simulink model "Project2_2"  (R2025b)
settings: Solver=VariableStepAuto  StartTime=0.0  StopTime=10.0  RelTol=1e-3
undefined symbols (not defined in the file or in its folder): A, F, Ti
settings Model: Creator=night  LastModifiedBy=night

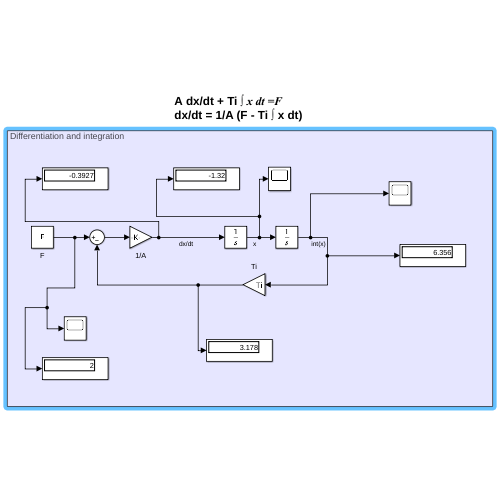
[thumbnail: Simulink's stored preview of the top-level diagram]
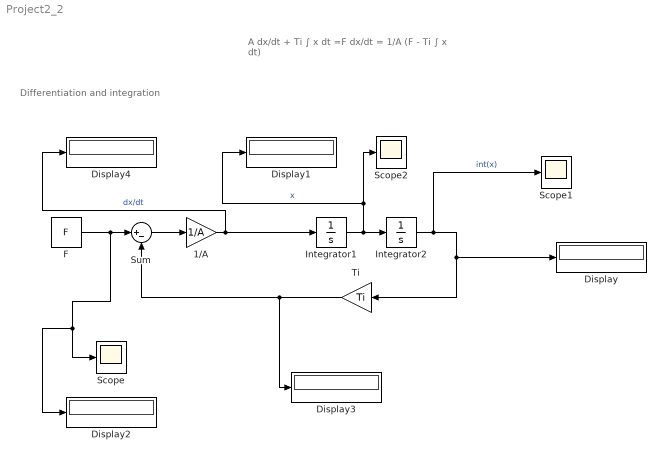
== system Project2_2 ==
  note: A dx/dt + Ti ∫ x dt =F
      | dx/dt = 1/A (F - Ti ∫ x dt)
  note: Differentiation and integration
  1/A : Gain  Gain=1/A
  Display{,1..4} (5 alike) : Display
  F : Constant  Value=F
  Integrator1 : Integrator
  Integrator2 : Integrator
  Scope : Scope
      settings: ActiveDisplayYMinimum=1  ActiveDisplayYMaximum=3
  Scope1 : Scope
      settings: ActiveDisplayYMinimum=-1  ActiveDisplayYMaximum=1
  Scope2 : Scope
      settings: ActiveDisplayYMinimum=-1  ActiveDisplayYMaximum=1  DataLoggingVariableName=ScopeData2
  Sum : Sum  Inputs=|+-
  Ti : Gain  Gain=Ti
  wires:
  Ti/1 -> Display3/1, Sum/2
  1/A/1 -> Display4/1, Integrator1/1  "dx/dt"
  Integrator2/1 -> Scope1/1, Display/1, Ti/1  "int(x)"
  F/1 -> Display2/1, Scope/1, Sum/1
  Sum/1 -> 1/A/1
  Integrator1/1 -> Display1/1, Scope2/1, Integrator2/1  "x"
